simulink model "linear_ode_model"  (R2024a)
settings: Solver=ode45  StartTime=0  StopTime=5  MaxStep=0.01  RelTol=1e-3
undefined symbols (not defined in the file): DiscIntNeverNeededParam
settings Model: Creator=andrey  LastModifiedBy=andrey

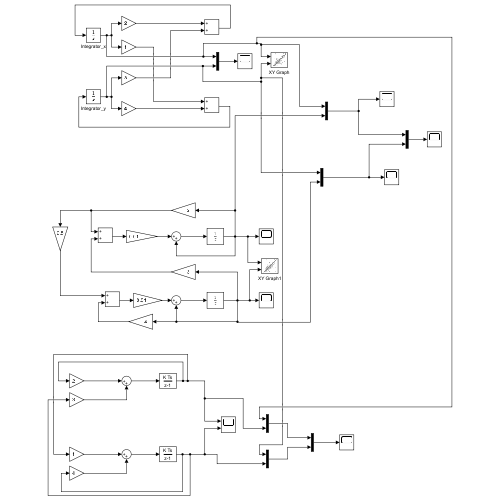
[thumbnail: Simulink's stored preview of the top-level diagram]
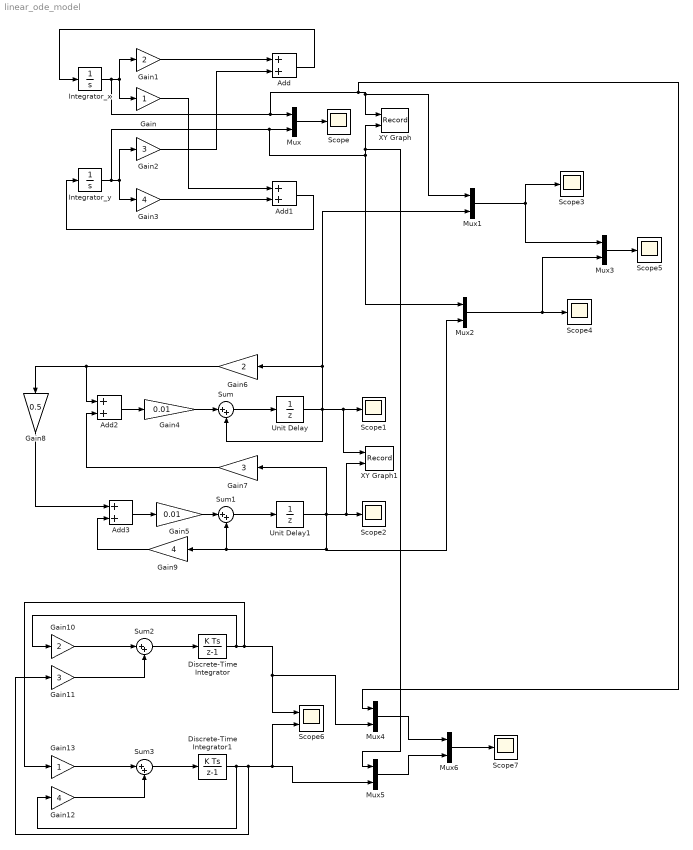
== system linear_ode_model ==
  Add{,1..3} (4 alike) : Sum
  Discrete-Time Integrator : DiscreteIntegrator  InitialCondition=1  SampleTime=-1  ICPrevOutput=DiscIntNeverNeededParam  ICPrevScaledInput=DiscIntNeverNeededParam
  Discrete-Time Integrator1 : DiscreteIntegrator  SampleTime=-1  ICPrevOutput=DiscIntNeverNeededParam  ICPrevScaledInput=DiscIntNeverNeededParam
  Gain : Gain
  Gain1 : Gain  Gain=2
  Gain10 : Gain  Gain=2
  Gain11 : Gain  Gain=3
  Gain12 : Gain  Gain=4
  Gain13 : Gain
  Gain2 : Gain  Gain=3
  Gain3 : Gain  Gain=4
  Gain4 : Gain  Gain=0.01
  Gain5 : Gain  Gain=0.01
  Gain6 : Gain  Gain=2
  Gain7 : Gain  Gain=3
  Gain8 : Gain  Gain=0.5
  Gain9 : Gain  Gain=4
  Integrator_x : Integrator  InitialCondition=1
  Integrator_y : Integrator
  Mux{,1..6} (7 alike) : Mux  Inputs=2
  Scope{,1..5,7} (7 alike) : Scope
  Scope6 : Scope  NumInputPorts=2
  Sum{,1..3} (4 alike) : Sum  Inputs=|++
  Unit Delay : UnitDelay  InitialCondition=1  SampleTime=-1  HasFrameUpgradeWarning=on
  Unit Delay1 : UnitDelay  SampleTime=-1  HasFrameUpgradeWarning=on
  XY Graph : Record  FileSettingsInternal="{\"entries\":[{\"content\":{\"excelSettings\":{\"content\":{},\"type\":\"Streamout.ExcelSettings\"}},\"type\":\"Streamout.FileSettingStorage\",\"uuid\":\"\"}],\"packageUris\":[\"http:\\/\\/schema.mathworks.com\\/mf0\\/streamout_blocks\\/R2020a\"],\"version\":\"1.0\"}"  Layout=[1 1]  SignalsInternal="{\"entries\":[{\"content\":{\"signals\":[{\"content\":{\"blockPath\":[],\"dimensions\":[1],\"domain\":\"\",\"lineColor\":\"#a2142f\",\"plots\":[ 1 ],\"port\":1,\"sid\":[\"\"],\"signalID\":1,\"signalName\":\"Integrator_x\"},\"type\":\"RecordBlkView.Signal\",\"uuid\":\"\"},{\"content\":{\"blockPath\":[],\"dimensions\":[1],\"domain\":\"\",\"lineColor\":\"#139fff\",\"plots\":[ 1 ],\"port\":2,\"sid\":[\"\"],\"signalID\":2,\"signalName\":\"Integrator_y\"},\"type\":\"RecordBlkView.Signal\",\"uuid\":\"\"}]},\"type\":\"RecordBlkView.InputSignals\",\"uuid\":\"\"}],\"packageUris\":[\"http:\\/\\/schema.mathworks.com\\/mf0\\/streamout_blocks\\/R2020a\"],\"version\":\"1.0\"}"  VisualizationBindings="{\"xyplotplugin\":{\"info\":[{\"series\":[{\"bindingParametersList\":[{\"parameter\":\"X-Axis\",\"signalID\":1,\"signalName\":\"Integrator_x\"},{\"parameter\":\"Y-Axis\",\"signalID\":2,\"signalName\":\"Integrator_y\"}],\"seriesID\":0}],\"subplotID\":1}]}}"  CompatibilityTag=XY
  XY Graph1 : Record  FileSettingsInternal="{\"entries\":[{\"content\":{\"excelSettings\":{\"content\":{},\"type\":\"Streamout.ExcelSettings\"}},\"type\":\"Streamout.FileSettingStorage\",\"uuid\":\"\"}],\"packageUris\":[\"http:\\/\\/schema.mathworks.com\\/mf0\\/streamout_blocks\\/R2020a\"],\"version\":\"1.0\"}"  Layout=[1 1]  SignalsInternal="{\"entries\":[{\"content\":{\"signals\":[{\"content\":{\"blockPath\":[],\"dimensions\":[1],\"domain\":\"\",\"lineColor\":\"#a2142f\",\"plots\":[ 1 ],\"port\":1,\"sid\":[\"\"],\"signalID\":1,\"signalName\":\"Unit Delay\"},\"type\":\"RecordBlkView.Signal\",\"uuid\":\"\"},{\"content\":{\"blockPath\":[],\"dimensions\":[1],\"domain\":\"\",\"lineColor\":\"#139fff\",\"plots\":[ 1 ],\"port\":2,\"sid\":[\"\"],\"signalID\":2,\"signalName\":\"Unit Delay1\"},\"type\":\"RecordBlkView.Signal\",\"uuid\":\"\"}]},\"type\":\"RecordBlkView.InputSignals\",\"uuid\":\"\"}],\"packageUris\":[\"http:\\/\\/schema.mathworks.com\\/mf0\\/streamout_blocks\\/R2020a\"],\"version\":\"1.0\"}"  VisualizationBindings="{\"xyplotplugin\":{\"info\":[{\"series\":[{\"bindingParametersList\":[{\"parameter\":\"X-Axis\",\"signalID\":1,\"signalName\":\"Unit Delay\"},{\"parameter\":\"Y-Axis\",\"signalID\":2,\"signalName\":\"Unit Delay1\"}],\"seriesID\":0}],\"subplotID\":1}]}}"  CompatibilityTag=XY
  wires:
  Integrator_x/1 -> Mux1/1, XY Graph/1, Mux4/1, Mux/1, Gain/1, Gain1/1
  Integrator_y/1 -> Mux5/1, XY Graph/2, Mux2/1, Mux/2, Gain3/1, Gain2/1
  Gain1/1 -> Add/1
  Gain2/1 -> Add/2
  Add/1 -> Integrator_x/1
  Gain/1 -> Add1/1
  Gain3/1 -> Add1/2
  Add1/1 -> Integrator_y/1
  Mux/1 -> Scope/1
  Unit Delay/1 -> XY Graph1/1, Scope1/1, Sum/2, Mux1/2, Gain6/1
  Unit Delay1/1 -> Mux2/2, Gain9/1, Sum1/2, Gain7/1, XY Graph1/2, Scope2/1
  Sum1/1 -> Unit Delay1/1
  Sum/1 -> Unit Delay/1
  Gain5/1 -> Sum1/1
  Gain4/1 -> Sum/1
  Gain6/1 -> Gain8/1, Add2/1
  Gain7/1 -> Add2/2
  Add2/1 -> Gain4/1
  Add3/1 -> Gain5/1
  Gain8/1 -> Add3/1
  Gain9/1 -> Add3/2
  Mux1/1 -> Mux3/1, Scope3/1
  Mux2/1 -> Mux3/2, Scope4/1
  Mux3/1 -> Scope5/1
  Discrete-Time Integrator/1 -> Mux4/2, Scope6/1, Gain13/1, Gain10/1
  Sum2/1 -> Discrete-Time Integrator/1
  Gain10/1 -> Sum2/1
  Gain11/1 -> Sum2/2
  Discrete-Time Integrator1/1 -> Scope6/2, Mux5/2, Gain11/1, Gain12/1
  Gain13/1 -> Sum3/1
  Gain12/1 -> Sum3/2
  Sum3/1 -> Discrete-Time Integrator1/1
  Mux4/1 -> Mux6/1
  Mux5/1 -> Mux6/2
  Mux6/1 -> Scope7/1
